simulink model "scars_pwsat2_backup"  (R2019b)
settings: Solver=ode14x  StartTime=0.0  StopTime=40*24*60*60  FixedStep=10  RelTol=1e-3
values from neighbouring files (symbols this model uses):
  initEuler = [0 0 0]    [SCARSSetup.m]    (also in pwsat2_setup.m; scars_setup.m)
undefined symbols (not defined in the file or in its folder): Earth, WGS84
libraries: scars_library x3, aerolibutil x2, aerolib6dof2 x1, sharedtransform x1
settings Model: Creator=asmialek  LastModifiedBy=asmialek
settings DataIOCC: ReturnWorkspaceOutputsName=scars_out

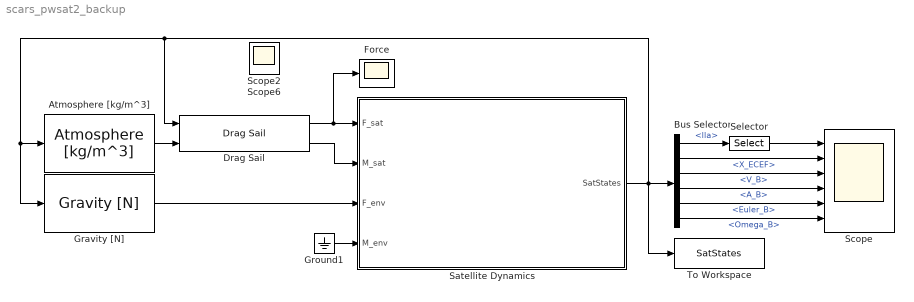
== system scars_pwsat2_backup ==
  Atmosphere [kg/m^3] : scars_library/Environment/Atmosphere [kg//m^3]  SystemSampleTime=-1  Latency=0  AutoFrameSizeCalculation=off
  Bus Selector : BusSelector  OutputSignals=lla,X_ECEF,V_B,A_B,Euler_B,Omega_B
  Drag Sail : scars_library/Actuators/Drag Sail  area_vector=[4 0 0]  C_d=[1 1 1]  ds_time=25.3*24*60*60  ds_duration=100  ds_moments=[0.5e-5 0.3e-5 1.7e-5]
  Force : Scope
  Gravity [N] : scars_library/Environment/Gravity [N]  mass=2.5
  Ground1 : Ground
  Satellite Dynamics : Subsystem  AncestorBlock=scars_library/Advanced/Satellite Dynamics
      mask Display: image('pw-sat-2__2.jpg'); % Use "Edit Image" on toolstrip to change.
  Scope : Scope  NumInputPorts=6
  Selector : Selector  InputPortWidth=3  IndexOptions=Index vector (dialog)  Indices=3  OutputSizes=1
  To Workspace : ToWorkspace  VariableName=SatStates  SaveFormat=Timeseries  SampleTime=-1
  Scope2 : Scope
  Scope6 : Scope
  wires:
  Ground1/1 -> Satellite Dynamics/4(M_env)
  Bus Selector/2 -> Scope/2  "<X_ECEF>"
  Gravity [N]/1 -> Satellite Dynamics/3(F_env)
  Drag Sail/1 -> Force/1, Satellite Dynamics/1(F_sat)
  Atmosphere [kg/m^3]/1 -> Drag Sail/2
  Bus Selector/1 -> Selector/1  "<lla>"
  Selector/1 -> Scope/1
  Satellite Dynamics/1(SatStates) -> Drag Sail/1, Gravity [N]/1, Atmosphere [kg/m^3]/1, To Workspace/1, Bus Selector/1
  Bus Selector/3 -> Scope/3  "<V_B>"
  Bus Selector/4 -> Scope/4  "<A_B>"
  Bus Selector/5 -> Scope/5  "<Euler_B>"
  Bus Selector/6 -> Scope/6  "<Omega_B>"
  Drag Sail/2 -> Satellite Dynamics/2(M_sat)

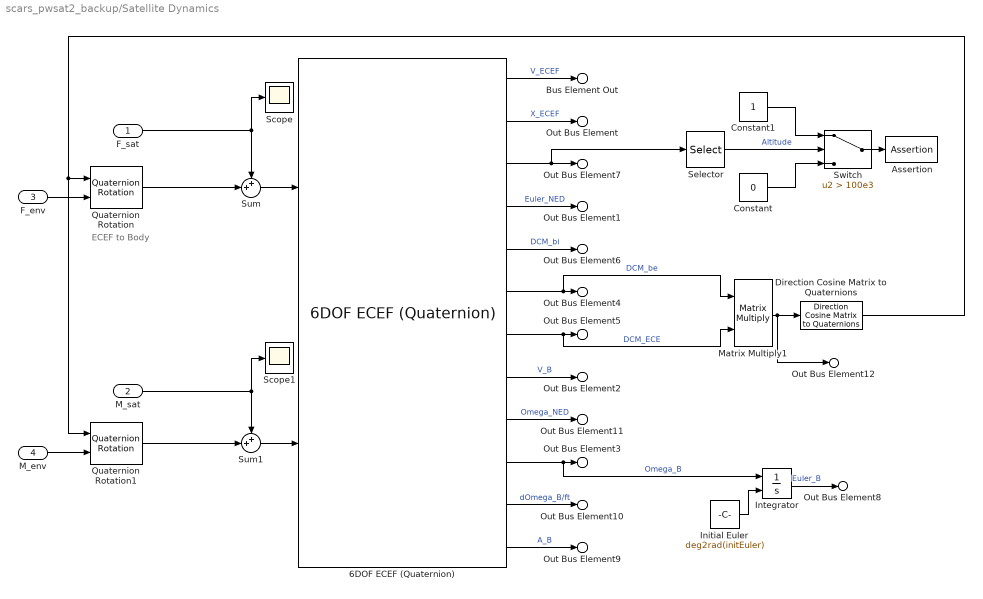
== system scars_pwsat2_backup/Satellite Dynamics ==
  note: ECEF to Body
  F_sat : Inport
  M_sat : Inport  Port=2
  F_env : Inport  Port=3
  M_env : Inport  Port=4
  6DOF ECEF (Quaternion) : aerolib6dof2/6DOF ECEF (Quaternion)  units=Metric (MKS)  mtype=Fixed  xg_0=r_lla  Vm_0=v_b  eul_0=deg2rad(initEuler)  pm_0=initEulerRates  mass_0=2.5  mass_e=0.5  mass_f=2.0  inertia=eye(3)  inertia_e=eye(3)  inertia_f=2*eye(3)  vre_flag=on  abi_flag=off  ptype=Earth (WGS84)  R=6378137  F=1/298.257223563  w_E=7292115e-11  angle_in=Internal  LG0=0  quat_statename=''  pm_statename=''  Vm_statename=''  posECEF_statename=''  posECI_statename=''  LG_statename=''  mass_statename=''
      settings: SourceProductName=Aerospace Blockset  SourceProductBaseCode=AE
  Assertion : Assertion
  Constant : Constant  Value=0
  Constant1 : Constant
  Direction Cosine Matrix to Quaternions : sharedtransform/Direction Cosine Matrix  to Quaternions  aMode=0  action=None  tolerance=eps(2)
      settings: SourceProductName=Aerospace Blockset  SourceProductBaseCode=AE
  Initial Euler : Constant  Value=deg2rad(initEuler)
  Integrator : Integrator  InitialConditionSource=external  WrapState=on
  Matrix Multiply1 : Product  Multiplication=Matrix(*)
  Quaternion Rotation : aerolibutil/Quaternion Rotation
  Quaternion Rotation1 : aerolibutil/Quaternion Rotation
  Scope : Scope
  Scope1 : Scope
  Selector : Selector  InputPortWidth=3  IndexOptions=Index vector (dialog)  Indices=3  OutputSizes=1
  Sum : Sum  Inputs=++|
  Sum1 : Sum  Inputs=++|
  Switch : Switch  Criteria=u2 > Threshold  Threshold=100e3
  Bus Element Out : Outport  PortName=SatStates  Element=V_ECEF
  Out Bus Element : Outport  PortName=SatStates  Element=X_ECEF
  Out Bus Element1 : Outport  PortName=SatStates  Element=Euler_NED
  Out Bus Element2 : Outport  PortName=SatStates  Element=V_B
  Out Bus Element3 : Outport  PortName=SatStates  Element=Omega_B
  Out Bus Element6 : Outport  PortName=SatStates  Element=DCM_ECI2B
  Out Bus Element4 : Outport  PortName=SatStates  Element=DCM_NED2B
  Out Bus Element5 : Outport  PortName=SatStates  Element=DCM_ECEF2NED
  Out Bus Element7 : Outport  PortName=SatStates  Element=lla
  Out Bus Element8 : Outport  PortName=SatStates  Element=Euler_B
  Out Bus Element9 : Outport  PortName=SatStates  Element=A_B
  Out Bus Element10 : Outport  PortName=SatStates  Element=dOmega_B/dt
  Out Bus Element11 : Outport  PortName=SatStates  Element=Omega_NED
  Out Bus Element12 : Outport  PortName=SatStates  Element=DCM_ECEF2B
  wires:
  Constant/1 -> Switch/3
  6DOF ECEF (Quaternion)/9 -> Out Bus Element11/1  "Omega_NED"
  Initial Euler/1 -> Integrator/2
  M_env/1 -> Quaternion Rotation1/2
  6DOF ECEF (Quaternion)/12 -> Out Bus Element9/1  "A_B"
  6DOF ECEF (Quaternion)/7 -> Matrix Multiply1/2, Out Bus Element5/1  "DCM_ECE"
  6DOF ECEF (Quaternion)/11 -> Out Bus Element10/1  "dOmega_B/ft"
  6DOF ECEF (Quaternion)/3 -> Selector/1, Out Bus Element7/1
  6DOF ECEF (Quaternion)/5 -> Out Bus Element6/1  "DCM_bi"
  Sum/1 -> 6DOF ECEF (Quaternion)/1
  Integrator/1 -> Out Bus Element8/1  "Euler_B"
  F_env/1 -> Quaternion Rotation/2
  Direction Cosine Matrix to Quaternions/1 -> Quaternion Rotation1/1, Quaternion Rotation/1
  F_sat/1 -> Scope/1, Sum/1
  Quaternion Rotation/1 -> Sum/2
  Quaternion Rotation1/1 -> Sum1/2
  Sum1/1 -> 6DOF ECEF (Quaternion)/2
  Matrix Multiply1/1 -> Direction Cosine Matrix to Quaternions/1, Out Bus Element12/1
  6DOF ECEF (Quaternion)/1 -> Bus Element Out/1  "V_ECEF"
  Selector/1 -> Switch/2  "Altitude"
  6DOF ECEF (Quaternion)/4 -> Out Bus Element1/1  "Euler_NED"
  6DOF ECEF (Quaternion)/6 -> Matrix Multiply1/1, Out Bus Element4/1  "DCM_be"
  6DOF ECEF (Quaternion)/2 -> Out Bus Element/1  "X_ECEF"
  Switch/1 -> Assertion/1
  Constant1/1 -> Switch/1
  6DOF ECEF (Quaternion)/10 -> Integrator/1, Out Bus Element3/1  "Omega_B"
  6DOF ECEF (Quaternion)/8 -> Out Bus Element2/1  "V_B"
  M_sat/1 -> Sum1/1, Scope1/1
